simulink model "zad1"  (R2016a)
settings: Solver=VariableStepAuto  StartTime=0.0  StopTime=12  MaxStep=2^-7  RelTol=1e-3
settings Model: Creator=sk42595  LastModifiedBy=sk42595

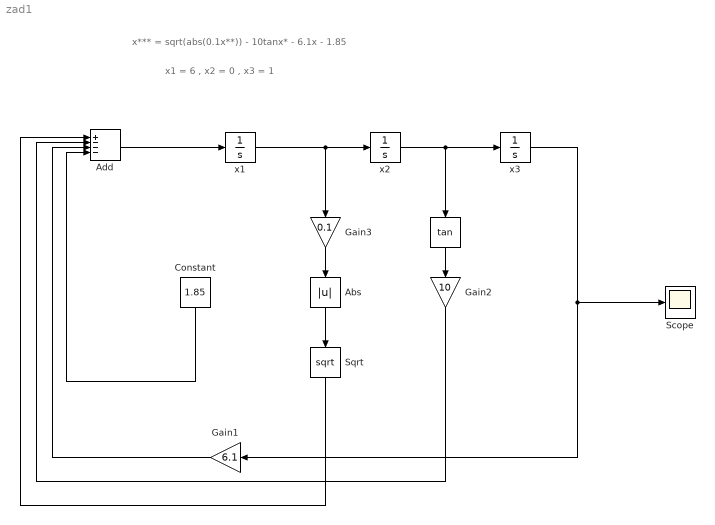
== system zad1 ==
  note: x1 = 6 , x2 = 0 , x3 = 1
  note: x*** = sqrt(abs(0.1x**)) - 10tanx* - 6.1x - 1.85
  " " : Trigonometry  Operator=tan
  Abs : Abs
  Add : Sum  Inputs=+---
  Constant : Constant  Value=1.85
  Gain1 : Gain  Gain=6.1
  Gain2 : Gain  Gain=10
  Gain3 : Gain  Gain=0.1
  Scope : Scope
  Sqrt : Sqrt  SaturateOnIntegerOverflow=on
  x1 : Integrator  InitialCondition=1
  x2 : Integrator
  x3 : Integrator  InitialCondition=6
  wires:
  Add/1 -> x1/1
  Constant/1 -> Add/4
  Gain1/1 -> Add/3
  x1/1 -> x2/1, Gain3/1
  x2/1 -> " "/1, x3/1
  x3/1 -> Scope/1, Gain1/1
  Sqrt/1 -> Add/1
  Gain3/1 -> Abs/1
  Abs/1 -> Sqrt/1
  " "/1 -> Gain2/1
  Gain2/1 -> Add/2
